simulink model "DASD_B_Project_3"  (R2025b)
settings: Solver=FixedStepAuto  StartTime=0.0  StopTime=200  FixedStep=0.01  RelTol=1e-3
values from neighbouring files (symbols this model uses):
  a = 0.923    [VehicleParameters.m]
  a_max_acc = 2.0    (= 2)    [main.m]
  a_max_dec = -3.5    [main.m]
  ABS_parameters = [lower_acc; lower_slip; higher_acc; mean_acc; rise_rate; fall_rate]    [main.m]
  b = 1.376    [VehicleParameters.m]
  CMy = 0.1    [VehicleParameters.m]
  coeff = ones(1, fir_window) / fir_window    [main.m]
  Cx = 0.33    [VehicleParameters.m]
  Cz = 0.2    [VehicleParameters.m]
  dist0 = 100    [main.m]
  eta_t = 0.93    [VehicleParameters.m]
  f0 = 0.011    [VehicleParameters.m]
  g = 9.81    [VehicleParameters.m]
  gear_vec = i_g    [main.m]
  h = 2.7    [main.m]
  hG = 0.6    [VehicleParameters.m]
  I = kp / tau_virtual    (= 1.66666666667)    [main.m]
  i_f = 3.438    [VehicleParameters.m]
  i_g = [3.909 , 2.157 , 1.48 , 1.121 , 0.897]    [VehicleParameters.m]
  Je = 0.088    [VehicleParameters.m]
  Jt = 0.05    [VehicleParameters.m]
  Jw = 0.59    [VehicleParameters.m]
  K = 2.6e-8    (= 2.6e-08)    [VehicleParameters.m]
  l = a+b    (= 2.299)    [VehicleParameters.m]
  lambda = 0.8    [main.m]
  m = 1020    [VehicleParameters.m]
  mu_vec = road_cond{choice}    [main.m]
  n_shiftdown = 200    [main.m]
  n_shiftup = 500    [main.m]
  n_vec = n_vec_set{vec_choice}    [main.m]
  omega0 = v0/Re    [main.m]
  P = kp    (= 0.333333333333)    [main.m]
  Rc = Re    (= 0.279)    [VehicleParameters.m]
  ro = 1.2    [VehicleParameters.m]
  S = 2.04    [VehicleParameters.m]
  sigma_vec = sigma    [main.m]
  startingGear = 3    [main.m]
  t_pedalAct = 0.8    [VehicleParameters.m]
  t_shifting = 0.2    [VehicleParameters.m]
  T_vec = T_vec_set{vec_choice}    [main.m]
  tau_f = 1./i_f    (= 0.290866783013)    [VehicleParameters.m]
  Tc_max = 1.2*Te_max    (= 126)    [VehicleParameters.m]
  Traction = 1    [VehicleParameters.m]
  Ts = 0.01    [main.m]
  v0 = 30    [main.m]
  v_min_acc = 5.0    (= 5)    [main.m]
  v_set_min = 7.0    (= 7)    [main.m]
libraries: simulink x29, slpidlib x1
(part 2 of 2)

== matlab function DASD_B_Project_3/Ego Vehicle/Wheel dynamics/FR wheel/MATLAB Function ==
  data: state input; T_brake input; slip input; params input; NextState output; omega_dot input; T_brake output
function [NextState, T_brake] = fcn(state, T_brake, slip, params, omega_dot)
%%% Next State represents the ABS valve condition at the next time step
%%% 1 = increase
%%% 2 = hold
%%% 3 = release
%%% 4 = hold
%%% 5 = increase
%%% 6 = hold
%%% 7 = increase less
%%% 8 = release (3)

lower_acc = params(1);
lower_slip = params(2);
higher_acc = params(3);
mean_acc = params(4);
rise_rate = params(5);
fall_rate = params(6);


switch state
    case 1
        if omega_dot < lower_acc
            NextState = 2;
        else
            NextState = 1;
        end
        T_brake = T_brake + rise_rate;
    case 2
        if slip < lower_slip
            NextState = 3;
        else
            NextState = 2;
        end
        T_brake = T_brake;
    case 3
        if slip > lower_slip
            NextState = 4;
        else
            NextState = 3;
        end
        T_brake = T_brake - fall_rate;
    case 4 
        if omega_dot > higher_acc
            NextState = 5;
        else
            NextState = 4;
        end
        T_brake = T_brake;
    case 5 
        if omega_dot < higher_acc
            NextState = 6;
        else
            NextState = 5;
        end
        T_brake = T_brake + rise_rate;
    case 6
        if omega_dot < mean_acc
            NextState = 7;
        else 
            NextState = 6;
        end
        T_brake = T_brake;
    case 7
        if omega_dot < lower_acc
            NextState = 3;
        else
            NextState = 7;
        end
        T_brake = T_brake + 0.5*rise_rate;
    otherwise
        NextState = state;
        T_brake = T_brake;
end
end

== matlab function DASD_B_Project_3/Ego Vehicle/Gear shifting logic/Gear shifting logic ==
  data: omega_t input; gearRatio output; gN_vect input; shiftspeed input; gear output; gearPrevious input
function [gearRatio, gear] = fcn(omega_t, gN_vect, shiftspeed, gearPrevious)
gearRatio = gN_vect(gearPrevious);
gear = gearPrevious;
    if ( omega_t*gearRatio > shiftspeed(1)) && gearPrevious < length(gN_vect)
    %if ( omega_w*gearRatio > shiftspeed(1)) && gearPrevious < length(gN_vect) %omega_t*gearRatio > shiftspeed(1) ||
        gear = gearPrevious+1;
        gearRatio = gN_vect(gear);
    elseif omega_t*gearRatio < shiftspeed(2) && gearPrevious > 1
        gear = gearPrevious-1;
        gearRatio = gN_vect(gear);
    end
end

== matlab function DASD_B_Project_3/Ego Vehicle/Gear shifting logic/MATLAB Function ==
  data: hc output; trigger input; t input; t_step input; tNext output; t_pedalAct input; t_shifting input
function [hc, tNext] = fcn(trigger,t, t_step,t_pedalAct, t_shifting)
tNext = t+t_step;
    if trigger
        tNext = 0;
        hc = 1;
    else
        hc = 1+1./(1+exp(15*(t-t_pedalAct/2)))-1./(1+exp(15*(t-t_shifting-3*t_pedalAct/2)));
    end
end

== matlab function DASD_B_Project_3/Triggered Subsystem/MATLAB Function ==
function fcn

disp('ACC failure. You rammed the vehicle in front.')

== matlab function DASD_B_Project_3/Ego Vehicle/Engine + clutch/Clutch1 ==
  data: u input; Tc output; Tcmax input; Temax input; hc input; ha input
function Tc = fcn(u, Tcmax, Temax, hc, ha)
Tc = ha*Temax;
if Temax < 0
    Tc = Temax;
end
if u > 0
    Tc = hc*Tcmax;
elseif u < 0
    Tc = -hc*Tcmax;
end
end

== matlab function DASD_B_Project_3/Ego Vehicle/Wheel dynamics/RL wheel/MATLAB Function ==
  data: state input; T_brake input; slip input; params input; NextState output; omega_dot input; T_brake output
function [NextState, T_brake] = fcn(state, T_brake, slip, params, omega_dot)
%%% Next State represents the ABS valve condition at the next time step
%%% 1 = increase
%%% 2 = hold
%%% 3 = release
%%% 4 = hold
%%% 5 = increase
%%% 6 = hold
%%% 7 = increase less
%%% 8 = release (3)

lower_acc = params(1);
lower_slip = params(2);
higher_acc = params(3);
mean_acc = params(4);
rise_rate = params(5);
fall_rate = params(6);


switch state
    case 1
        if omega_dot < lower_acc
            NextState = 2;
        else
            NextState = 1;
        end
        T_brake = T_brake + rise_rate;
    case 2
        if slip < lower_slip
            NextState = 3;
        else
            NextState = 2;
        end
        T_brake = T_brake;
    case 3
        if slip > lower_slip
            NextState = 4;
        else
            NextState = 3;
        end
        T_brake = T_brake - fall_rate;
    case 4 
        if omega_dot > higher_acc
            NextState = 5;
        else
            NextState = 4;
        end
        T_brake = T_brake;
    case 5 
        if omega_dot < higher_acc
            NextState = 6;
        else
            NextState = 5;
        end
        T_brake = T_brake + rise_rate;
    case 6
        if omega_dot < mean_acc
            NextState = 7;
        else 
            NextState = 6;
        end
        T_brake = T_brake;
    case 7
        if omega_dot < lower_acc
            NextState = 3;
        else
            NextState = 7;
        end
        T_brake = T_brake + 0.5*rise_rate;
    otherwise
        NextState = state;
        T_brake = T_brake;
end
end

== matlab function DASD_B_Project_3/Ego Vehicle/Wheel dynamics/RR wheel/MATLAB Function ==
  data: state input; T_brake input; slip input; params input; NextState output; omega_dot input; T_brake output
function [NextState, T_brake] = fcn(state, T_brake, slip, params, omega_dot)
%%% Next State represents the ABS valve condition at the next time step
%%% 1 = increase
%%% 2 = hold
%%% 3 = release
%%% 4 = hold
%%% 5 = increase
%%% 6 = hold
%%% 7 = increase less
%%% 8 = release (3)

lower_acc = params(1);
lower_slip = params(2);
higher_acc = params(3);
mean_acc = params(4);
rise_rate = params(5);
fall_rate = params(6);


switch state
    case 1
        if omega_dot < lower_acc
            NextState = 2;
        else
            NextState = 1;
        end
        T_brake = T_brake + rise_rate;
    case 2
        if slip < lower_slip
            NextState = 3;
        else
            NextState = 2;
        end
        T_brake = T_brake;
    case 3
        if slip > lower_slip
            NextState = 4;
        else
            NextState = 3;
        end
        T_brake = T_brake - fall_rate;
    case 4 
        if omega_dot > higher_acc
            NextState = 5;
        else
            NextState = 4;
        end
        T_brake = T_brake;
    case 5 
        if omega_dot < higher_acc
            NextState = 6;
        else
            NextState = 5;
        end
        T_brake = T_brake + rise_rate;
    case 6
        if omega_dot < mean_acc
            NextState = 7;
        else 
            NextState = 6;
        end
        T_brake = T_brake;
    case 7
        if omega_dot < lower_acc
            NextState = 3;
        else
            NextState = 7;
        end
        T_brake = T_brake + 0.5*rise_rate;
    otherwise
        NextState = state;
        T_brake = T_brake;
end
end

== matlab function DASD_B_Project_3/MATLAB Function ==
  data: a_target input; ha output; hb output; v input; tau_g input
function [ha, hb] = inverse_pedals(a_target, v, tau_g)
    % INVERSE_PEDALS Calculates the required accelerator and brake pedal positions.
    % 
    % This function determines the necessary accelerator (ha) and brake (hb)
    % commands to achieve a target acceleration, given the current vehicle
    % speed and gear ratio. It acts as the low-level controller for the ACC.
    %
    % INPUTS:
    %   a_target: Desired acceleration from the ACC controller [m/s^2]
    %   v:        Current vehicle speed [m/s]
    %   tau_g:    Transmission ratio of the currently engaged gear
    %
    % OUTPUTS:
    %   ha:       Accelerator pedal position command [0 to 1]
    %   hb:       Brake pedal position command [0 to 1]

    % VEHICLE PARAMETERS 
    % Sourced from the 'VehicleParameters.m' file.
    m = 1020;         % [kg] Vehicle mass
    Te_max = 105;     % [Nm] Maximum engine torque
    Tb_max = 300;     % [Nm] Maximum braking torque on the front axle (Tbf_max)
    Kb = 2.3;         % [-] Brake bias ratio (front/rear distribution parameter)
    Re = 0.279;       % [m] Tire rolling radius
    tau_t = 1/3.438;  % [-] Final drive ratio (driveline transmission ratio, tau_f)
    eta_t = 0.93;     % [-] Total transmission efficiency
    eta_g = 1;        % [-] Gearbox efficiency (assumed 100% if not specified otherwise)
    f0 = 0.011; 
    K = 2.6e-8; % [s^2/m^2]
    Je     = 0.088; % engine inertia [kg*m^2]

    Jt     = 0.05;  % transmission inertia [kg*m^2]
    Jw     = 0.59;  % single wheel inertia [kg*m^2]
    me = m + (4 * Jw)/(Re^2) + Jt/(Re^2 * tau_t^2) + Je/(Re^2 * tau_g^2 * tau_t^2);  % equivalent mass
    S      = 2.04;  % resistant area [m^2]
    Cx     = 0.33;  % drag coefficient
    Cz     = 0.2;   % lift coefficient
    ro     = 1.2;   % dry air density at 20°C [kg/m^3]

    % Aerodynamic and rolling resistance coefficients
    % F_res = A + B*v^2 + C*v^4
    alpha = 0;
    g = 9.81;
     
    A     = m*g*(f0*cos(alpha)+sin(alpha)); % [N] Constant rolling resistance component
    B     = m*g*K*cos(alpha)+0.5*ro*S*(Cx-Cz*f0); % [N/(m/s)^2] Linear term
    C     = -0.5*ro*S*K*Cz;  % [N/(m/s)^4] Aerodynamic drag component (0.5 * rho * S * Cx)

    % FORCE CALCULATIONS 
    
    % Calculate the total resistance force acting on the vehicle at the current speed
    F_res = A + B*(v^2) + C*(v^4); 
    
    % Calculate the total force required at the wheels to achieve the target acceleration.
    % Newton's second law: F_req - F_res = me * a_target  =>  F_req = me * a_target + F_res
    F_req = me * a_target + F_res; 
    
    % Calculate the maximum possible traction force at the wheels (at 100% throttle)
    F_mot_max = (Te_max * eta_g * eta_t) / (Re * tau_g * tau_t);
    
    % Calculate the maximum possible braking force at the wheels (at 100% brake)
    F_brk_max = (Tb_max / Re) * (1 + 1/Kb);

    % INVERSION LOGIC
    
    if F_req > 0
        % Traction Phase: The required force is positive.
        % The engine needs to provide torque to overcome resistance and achieve acceleration.
        % We calculate the required throttle percentage. The brake is not needed.
        ha = F_req / F_mot_max;
        hb = 0;
    else
        % Braking Phase: The required force is negative or zero.
        ha = 0;
        hb = -F_req / F_brk_max;
    end

end
